simulink model "verify_sfun_storage_heatexchanger2_mdl"  (Simulink 8.2)
settings: Solver=VariableStepDiscrete  StartTime=0.0  StopTime=1  MaxStep=1  RelTol=1e-3
libraries: carnot x1
settings Model: Creator=drhf  LastModifiedBy=drhf

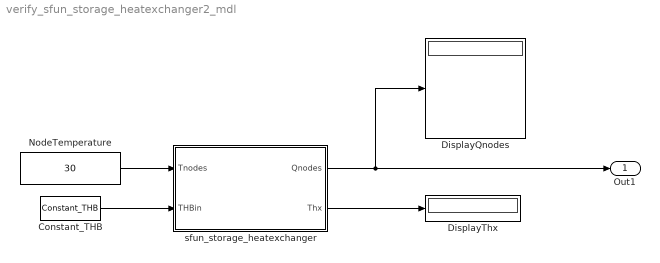
== system verify_sfun_storage_heatexchanger2_mdl ==
  Constant_THB : carnot/Source/Simple/Constant_THB  t=40  mdot=0.1  p=1e5  mID=No Pressure Drop  fluid=Water  mix=0  dia=0.02  hgt=0
  DisplayQnodes : Display
  DisplayThx : Display
  NodeTemperature : Constant  Value=30
  sfun_storage_heatexchanger : Subsystem  mask(storage heat exchanger){idn=heat transfer data fit EN12977  - stratified, nodes=1, inlet=1, outlet=1, pp=[ 102.7         0.226          0.55             0             0             0             0 ]}
      mask prompts: idn "type"; nodes "number of nodes"; inlet "inlet node"; outlet "outlet node"; pp "parameter vector"
      mask init:
      | switch(idn)
      |     case 1
      |         id = 201;
      |     case 2
      |         id = 301;
      |     case 3
      |         id = 202;
      |     case 4
      |         id = 302;
      |     case 5
      |         id = 203;
      |     case 6
      |         id = 303;
      |     case 7
      |         id = 204;
      |     case 8
      |         id = 304;
      | end
      mask TypeOptions idn: smooth tube theoretical | smooth tube theoretical - stratified | finned tube theoretical | finned tube theoretical  - stratified | heat transfer from data fit | heat transfer from data fit  - stratified | heat transfer data fit EN12977 | heat transfer data fit EN12977  - stratified
  Out1 : Outport
  wires:
  NodeTemperature/1 -> sfun_storage_heatexchanger/1(Tnodes)
  sfun_storage_heatexchanger/1(Qnodes) -> DisplayQnodes/1, Out1/1
  sfun_storage_heatexchanger/2(Thx) -> DisplayThx/1
  Constant_THB/1 -> sfun_storage_heatexchanger/2(THBin)

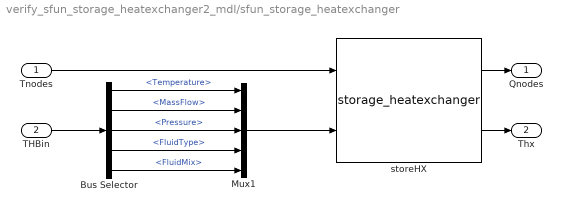
== system verify_sfun_storage_heatexchanger2_mdl/sfun_storage_heatexchanger ==
  Tnodes : Inport
  THBin : Inport  Port=2
  Bus Selector : BusSelector  OutputSignals=Temperature,MassFlow,Pressure,FluidType,FluidMix
  Mux1 : Mux  Inputs=5
  storeHX : S-Function  FunctionName=storage_heatexchanger  Parameters=id, nodes, inlet, outlet, pp(1), pp(2), pp(3), pp(4), pp(5), pp(6), pp(7)  EnableBusSupport=off
  Qnodes : Outport
  Thx : Outport  Port=2
  wires:
  storeHX/2 -> Thx/1
  THBin/1 -> Bus Selector/1
  storeHX/1 -> Qnodes/1
  Tnodes/1 -> storeHX/1
  Bus Selector/1 -> Mux1/1  "<Temperature>"
  Bus Selector/2 -> Mux1/2  "<MassFlow>"
  Bus Selector/3 -> Mux1/3  "<Pressure>"
  Bus Selector/4 -> Mux1/4  "<FluidType>"
  Bus Selector/5 -> Mux1/5  "<FluidMix>"
  Mux1/1 -> storeHX/2
